simulink library "getHomingGait"  (R2016b)
settings: Solver=VariableStepAuto  StartTime=0.0  StopTime=10.0  RelTol=1e-3
libraries: VariousLibrary x6, PositionSmoothener x1
settings Model: Creator=Taeke  LastModifiedBy=Taeke

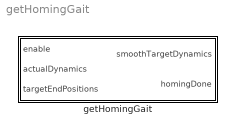
== system getHomingGait ==
  getHomingGait : Subsystem

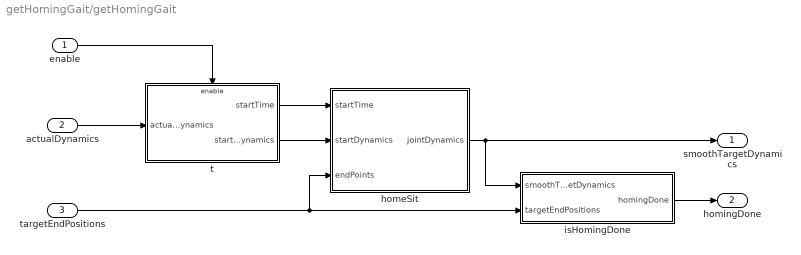
== system getHomingGait/getHomingGait ==
  enable : Inport
  actualDynamics : Inport  Port=2
  targetEndPositions : Inport  Port=3
  homeSit : Subsystem
  isHomingDone : Subsystem
  t : Subsystem
  smoothTargetDynamics : Outport
  homingDone : Outport  Port=2
  wires:
  isHomingDone/1(homingDone) -> homingDone/1
  actualDynamics/1 -> t/1(actualDynamics)
  targetEndPositions/1 -> isHomingDone/2(targetEndPositions), homeSit/3(endPoints)
  t/1(startTime) -> homeSit/1(startTime)
  t/2(startDynamics) -> homeSit/2(startDynamics)
  enable/1 -> t/Enable
  homeSit/1(jointDynamics) -> smoothTargetDynamics/1, isHomingDone/1(smoothTargetDynamics)

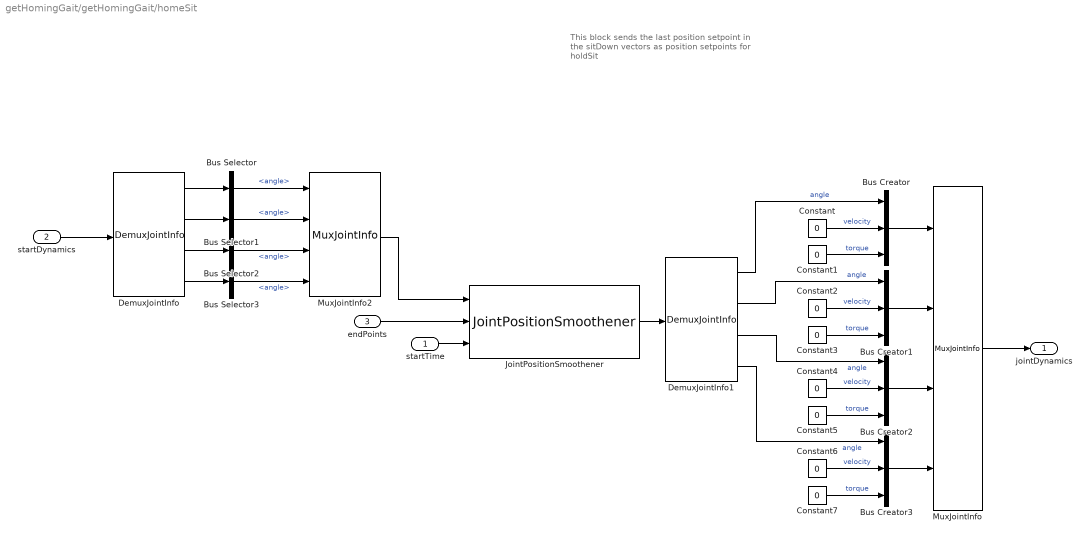
== system getHomingGait/getHomingGait/homeSit ==
  note: This block sends the last position setpoint
      | in the sitDown vectors as position setpoints
      | for holdSit
  startTime : Inport
  startDynamics : Inport  Port=2
  endPoints : Inport  Port=3
  Bus Creator{,1..3} (4 alike) : BusCreator  Inputs=3  OutDataTypeStr=Bus: JointDynamics  NonVirtualBus=on
  Bus Selector{,1..3} (4 alike) : BusSelector  OutputSignals=angle
  Constant{,1..7} (8 alike) : Constant  Value=0
  DemuxJointInfo : VariousLibrary/DemuxJointInfo
  DemuxJointInfo1 : VariousLibrary/DemuxJointInfo
  JointPositionSmoothener : PositionSmoothener/JointPositionSmoothener
  MuxJointInfo : VariousLibrary/MuxJointInfo
  MuxJointInfo2 : VariousLibrary/MuxJointInfo
  jointDynamics : Outport  OutDataTypeStr=Bus: JointDynamics
  wires:
  endPoints/1 -> JointPositionSmoothener/2
  JointPositionSmoothener/1 -> DemuxJointInfo1/1
  startTime/1 -> JointPositionSmoothener/3
  MuxJointInfo2/1 -> JointPositionSmoothener/1
  Bus Selector2/1 -> MuxJointInfo2/3  "<angle>"
  Bus Selector3/1 -> MuxJointInfo2/4  "<angle>"
  Bus Selector1/1 -> MuxJointInfo2/2  "<angle>"
  Bus Selector/1 -> MuxJointInfo2/1  "<angle>"
  DemuxJointInfo/2 -> Bus Selector1/1
  DemuxJointInfo/4 -> Bus Selector3/1
  DemuxJointInfo/3 -> Bus Selector2/1
  DemuxJointInfo/1 -> Bus Selector/1
  startDynamics/1 -> DemuxJointInfo/1
  DemuxJointInfo1/3 -> Bus Creator2/1  "angle"
  DemuxJointInfo1/2 -> Bus Creator1/1  "angle"
  DemuxJointInfo1/1 -> Bus Creator/1  "angle"
  Bus Creator3/1 -> MuxJointInfo/4
  Constant7/1 -> Bus Creator3/3  "torque"
  Constant6/1 -> Bus Creator3/2  "velocity"
  Bus Creator2/1 -> MuxJointInfo/3
  Constant5/1 -> Bus Creator2/3  "torque"
  Constant4/1 -> Bus Creator2/2  "velocity"
  Bus Creator1/1 -> MuxJointInfo/2
  Constant3/1 -> Bus Creator1/3  "torque"
  Constant2/1 -> Bus Creator1/2  "velocity"
  Bus Creator/1 -> MuxJointInfo/1
  Constant1/1 -> Bus Creator/3  "torque"
  Constant/1 -> Bus Creator/2  "velocity"
  MuxJointInfo/1 -> jointDynamics/1
  DemuxJointInfo1/4 -> Bus Creator3/1  "angle"

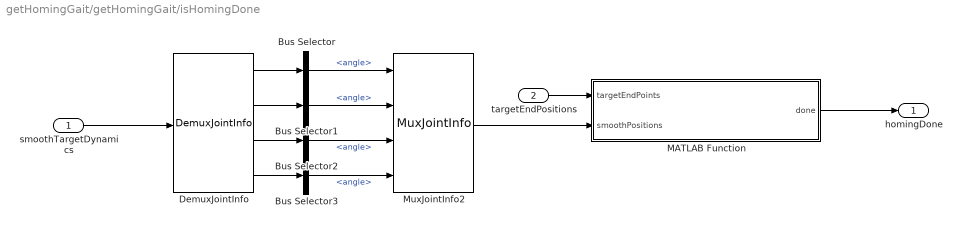
== system getHomingGait/getHomingGait/isHomingDone ==
  smoothTargetDynamics : Inport
  targetEndPositions : Inport  Port=2
  Bus Selector{,1..3} (4 alike) : BusSelector  OutputSignals=angle
  DemuxJointInfo : VariousLibrary/DemuxJointInfo
  MATLAB Function : MATLAB Function  TreatAsAtomicUnit=on
  MuxJointInfo2 : VariousLibrary/MuxJointInfo
  homingDone : Outport
  wires:
  MATLAB Function/1(done) -> homingDone/1
  targetEndPositions/1 -> MATLAB Function/1(targetEndPoints)
  MuxJointInfo2/1 -> MATLAB Function/2(smoothPositions)
  smoothTargetDynamics/1 -> DemuxJointInfo/1
  Bus Selector2/1 -> MuxJointInfo2/3  "<angle>"
  Bus Selector3/1 -> MuxJointInfo2/4  "<angle>"
  Bus Selector1/1 -> MuxJointInfo2/2  "<angle>"
  Bus Selector/1 -> MuxJointInfo2/1  "<angle>"
  DemuxJointInfo/2 -> Bus Selector1/1
  DemuxJointInfo/4 -> Bus Selector3/1
  DemuxJointInfo/3 -> Bus Selector2/1
  DemuxJointInfo/1 -> Bus Selector/1

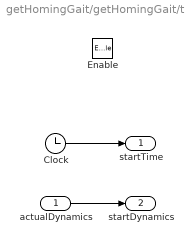
== system getHomingGait/getHomingGait/t ==
  actualDynamics : Inport
  Enable : EnablePort
  Clock : Clock
  startTime : Outport
  startDynamics : Outport  Port=2
  wires:
  actualDynamics/1 -> startDynamics/1
  Clock/1 -> startTime/1

== matlab function getHomingGait/isHomingDone/MATLAB Function ==
  data: targetEndPoints input; done output; smoothPositions input
function done = isHomingDone(targetEndPoints, smoothPositions)
done = all(abs(targetEndPoints - smoothPositions) < 0.01/360*2*pi); % we don't care about differences this small
end
